simulink model "pam_sys"  (R2019b)
settings: Solver=VariableStepAuto  StartTime=0.0  StopTime=10.0  RelTol=1e-3
libraries: commutil2 x4, commsink2 x2, commdigbbndam3 x2, commchan3 x1, commrandsrc3 x1
settings Model: Creator=yango  LastModifiedBy=yango

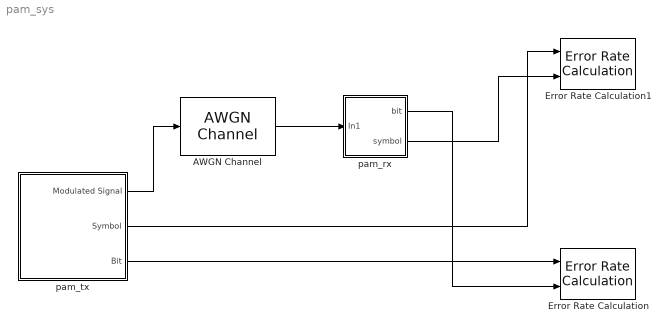
== system pam_sys ==
  AWGN Channel : commchan3/AWGN Channel  InputProcessing=Columns as channels (frame based)  seed=67  noiseMode="Signal to noise ratio  (Eb/No)"  EbNodB=SNR  EsNodB=10  SNRdB=10  bitsPerSym=1  Ps=5  Tsym=1/100000  variance=1
      settings: SourceProductName=Communications Toolbox
  Error Rate Calculation : commsink2/Error Rate Calculation  N=0  st_delay=0  cp_mode=Entire frame  subframe=[]  PMode=Workspace  WsName=BER  RsMode2=off  stop=off  numErr=100  maxBits=1e6
      settings: SourceProductName=Communications Toolbox
  Error Rate Calculation1 : commsink2/Error Rate Calculation  N=0  st_delay=0  cp_mode=Entire frame  subframe=[]  PMode=Workspace  WsName=SER  RsMode2=off  stop=off  numErr=100  maxBits=1e6
      settings: SourceProductName=Communications Toolbox
  "pam_rx " : Subsystem
  pam_tx : Subsystem
  wires:
  pam_tx/3(Bit) -> Error Rate Calculation/1
  pam_tx/1(Modulated Signal) -> AWGN Channel/1
  AWGN Channel/1 -> "pam_rx "/1(In1)
  "pam_rx "/1("bit ") -> Error Rate Calculation/2
  pam_tx/2(Symbol) -> Error Rate Calculation1/1
  "pam_rx "/2(symbol) -> Error Rate Calculation1/2

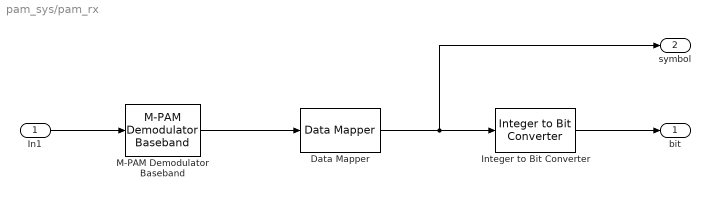
== system pam_sys/pam_rx  ==
  In1 : Inport
  Data Mapper : commutil2/Data Mapper  MapMode=Binary to Gray  M=4  MapVec=[0 1 3 2 7 6 4 5]
      settings: SourceProductName=Communications Toolbox  SourceProductBaseCode=CM
  Integer to Bit Converter : commutil2/Integer to Bit Converter  nbits=2  signedInputValues=Unsigned  bitOrder=MSB first  outDtype=Inherit via internal rule
      settings: SourceProductName=Communications Toolbox
  M-PAM Demodulator Baseband : commdigbbndam3/M-PAM Demodulator Baseband  M=4  OutType=Integer  Dec=Gray  PowType=Min. distance between symbols  MinDist=2  AvgPow=1  PeakPow=1  outDtype1=Inherit via internal rule  outDtype2=Inherit via internal rule  denormFactorWordLen=16  denormFactorDataTypeStr=Inherit: Same word length as input  denormFactorLastDataTypeStr=Inherit: Same word length as input  prodOutWordLen=16  prodOutRoundingMode=Floor  prodOutOverflowMode=Wrap  prodOutOvFlMode=off  prodOutOvFlModeLastStrValue=off  sumWordLen=16
      settings: SourceProductName=Communications Toolbox  SourceProductBaseCode=CM
  "bit " : Outport
  symbol : Outport  Port=2
  wires:
  In1/1 -> M-PAM Demodulator Baseband/1
  M-PAM Demodulator Baseband/1 -> Data Mapper/1
  Integer to Bit Converter/1 -> "bit "/1
  Data Mapper/1 -> symbol/1, Integer to Bit Converter/1

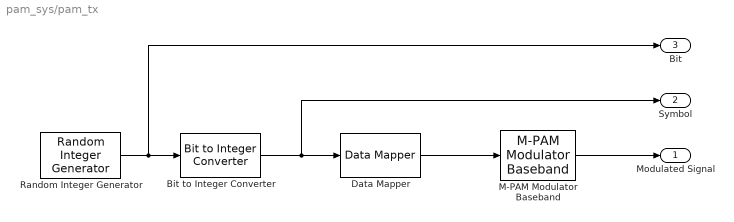
== system pam_sys/pam_tx ==
  Bit to Integer Converter : commutil2/Bit to Integer Converter  nbits=2  bitOrder=MSB first  signedOutputValues=Unsigned  outDtype=Inherit via internal rule  outDtypeSigned=Inherit via internal rule
      settings: SourceProductName=Communications Toolbox
  Data Mapper : commutil2/Data Mapper  MapMode=Binary to Gray  M=4  MapVec=[0 1 3 2 7 6 4 5]
      settings: SourceProductName=Communications Toolbox  SourceProductBaseCode=CM
  M-PAM Modulator Baseband : commdigbbndam3/M-PAM Modulator Baseband  M=4  InType=Integer  Enc=Gray  PowType=Min. distance between symbols  MinDist=2  AvgPow=1  PeakPow=1  outDtype=double  outWordLen=16  outUDDataType=sfix(16)  outFracLenMode=Best precision  outFracLen=15  outDataTypeStr=double  outLastDataTypeStr=double
      settings: SourceProductName=Communications Toolbox  SourceProductBaseCode=CM
  Random Integer Generator : commrandsrc3/Random Integer Generator  SetSize=2  SeedSource=Auto  Seed=0  SampleTime=1/200000  SamplesPerFrame=200000  OutputDataType=double  SimulateUsing=Interpreted execution
      settings: SourceProductName=Communications Toolbox
  Modulated Signal : Outport
  Symbol : Outport  Port=2
  Bit : Outport  Port=3
  wires:
  Bit to Integer Converter/1 -> Symbol/1, Data Mapper/1
  M-PAM Modulator Baseband/1 -> Modulated Signal/1
  Random Integer Generator/1 -> Bit/1, Bit to Integer Converter/1
  Data Mapper/1 -> M-PAM Modulator Baseband/1
